simulink model "distillation_example_1"  (R2024a)
settings: Solver=VariableStepAuto  StartTime=0.0  StopTime=10.0  RelTol=1e-3
settings Model: Creator=Braan  LastModifiedBy=Braan

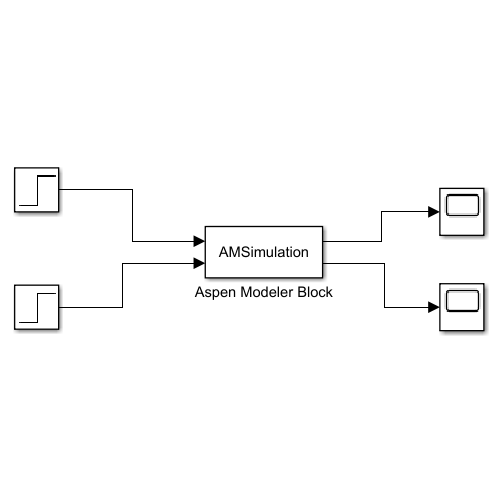
[thumbnail: Simulink's stored preview of the top-level diagram]
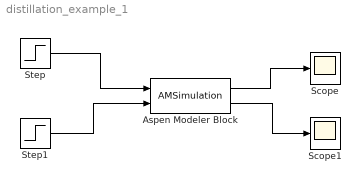
== system distillation_example_1 ==
  Aspen Modeler Block : M-S-Function  LoadFcn=|  FunctionName=AMSimulation  Parameters="'C:\\Users\\Braan\\OneDrive - NTNU\\10_V2024\\Master\\Distillation\\sim1_matlab.dynf','AD Application',2,'BLOCKS(\"COLUMN\").QRebR|MMkcal/hr\\BLOCKS(\"COLUMN\").Reflux.FmR|kg/hr',2,'STREAMS(\"D\").Zn(\"METHANOL\")|kmol/kmol\\STREAMS(\"B\").Zn(\"WATER\")|kmol/kmol',true,true,false"
      | LoadModel=actxserver('AMSimulation.Control');                 
      | invoke(LoadModel,'LoadModel',get_param(gcb,'Parameters'),pwd);
      | LoadModel.delete;
      | rehash;
      settings: DeleteFcn=|
      | CloseModel=actxserver('AMSimulation.Control');
      | invoke(CloseModel,'CloseModel',get_param(gcb,'Parameters'));
      | CloseModel.delete;
      settings: OpenFcn=|
      | SetupGUI=actxserver('AMSimulation.Setup');
      | NewParam=invoke(SetupGUI,'SetupModel',get_param(gcb,'Parameters'),pwd,get_param(gcb,'Name'));
      | set_param(gcb,'Parameters',NewParam);
      | SetupGUI.delete;
  Scope : Scope
  Scope1 : Scope
  Step : Step  Time=5  Before=1.042682977841136  After=2  SampleTime=0
  Step1 : Step  Time=8  Before=1464.968371888  After=2900  SampleTime=0
  wires:
  Aspen Modeler Block/1 -> Scope/1
  Aspen Modeler Block/2 -> Scope1/1
  Step/1 -> Aspen Modeler Block/1
  Step1/1 -> Aspen Modeler Block/2
